simulink model "observer"  (R2020b)
settings: Solver=VariableStepAuto  StartTime=0.0  StopTime=10.0  RelTol=1e-3
settings Model: Creator=10853  LastModifiedBy=10853

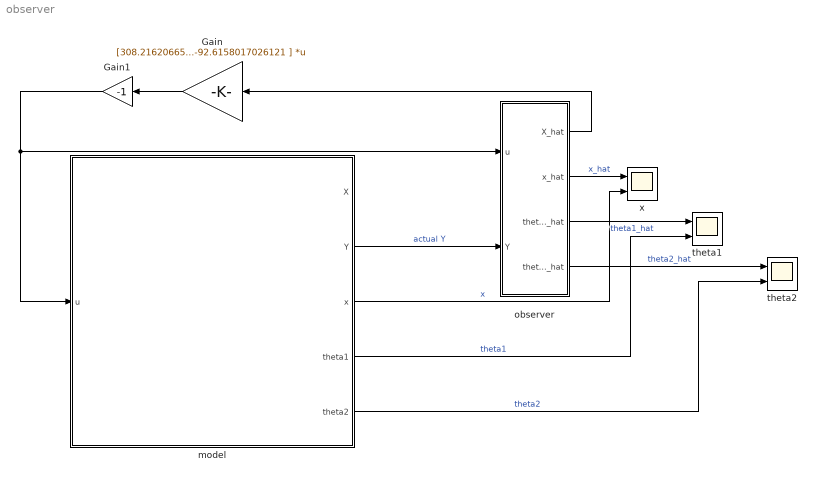
== system observer ==
  Gain : Gain  Gain=|  Multiplication=Matrix(K*u)
      | [308.216206651111	158.619423985671	-617.386289524257	151.829835967496	-19.2479620762821	-92.6158017026121
      | ]
  Gain1 : Gain  Gain=-1
  model : Subsystem
  observer : Subsystem
  theta1 : Scope  NumInputPorts=2
  theta2 : Scope  NumInputPorts=2
  x : Scope  NumInputPorts=2
  wires:
  model/3(x) -> x/2  "x"
  model/4(theta1) -> theta1/2  "theta1"
  model/2(Y) -> observer/2(Y)  "actual Y"
  Gain/1 -> Gain1/1
  Gain1/1 -> model/1(u), observer/1(u)
  observer/2(x_hat) -> x/1  "x_hat"
  observer/3(theta1_hat) -> theta1/1  "theta1_hat"
  model/5(theta2) -> theta2/2  "theta2"
  observer/4(theta2_hat) -> theta2/1  "theta2_hat"
  observer/1(X_hat) -> Gain/1

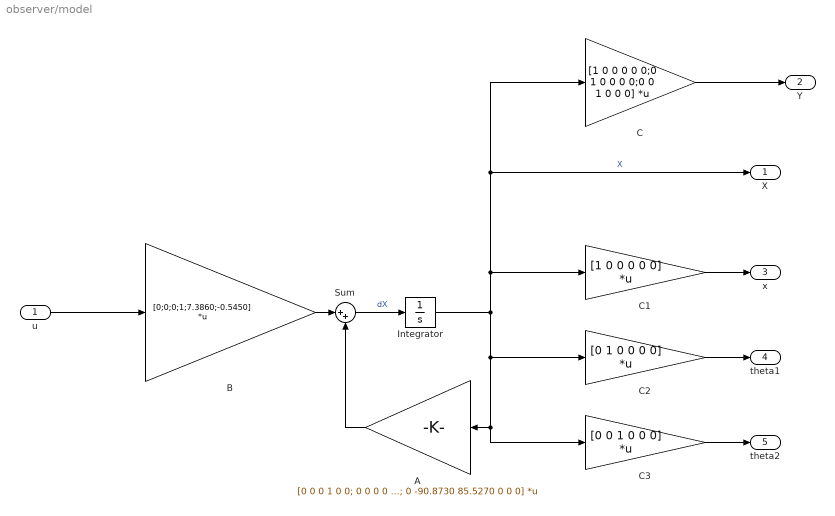
== system observer/model ==
  u : Inport
  A : Gain  Gain=[0 0 0 1 0 0; 0 0 0 0 1 0; 0 0 0 0 0 1;0 0 0 0 0 0; 0 189.318 -116.9320 0 0 0; 0 -90.8730 85.5270 0 0 0]  Multiplication=Matrix(K*u)
  B : Gain  Gain=[0;0;0;1;7.3860;-0.5450]  Multiplication=Matrix(K*u)
  C : Gain  Gain=[1 0 0 0 0 0;0 1 0 0 0 0;0 0 1 0 0 0]  Multiplication=Matrix(K*u)
  C1 : Gain  Gain=[1 0 0 0 0 0]  Multiplication=Matrix(K*u)
  C2 : Gain  Gain=[0 1 0 0 0 0]  Multiplication=Matrix(K*u)
  C3 : Gain  Gain=[0 0 1 0 0 0]  Multiplication=Matrix(K*u)
  Integrator : Integrator  InitialCondition=[0;pi/36;pi/36;0;0;0]
  Sum : Sum  Inputs=|++
  X : Outport
  Y : Outport  Port=2
  x : Outport  Port=3
  theta1 : Outport  Port=4
  theta2 : Outport  Port=5
  wires:
  u/1 -> B/1
  Integrator/1 -> C/1, X/1, C1/1, C2/1, C3/1, A/1  "X"
  C2/1 -> theta1/1
  B/1 -> Sum/1
  A/1 -> Sum/2
  Sum/1 -> Integrator/1  "dX"
  C1/1 -> x/1
  C3/1 -> theta2/1
  C/1 -> Y/1

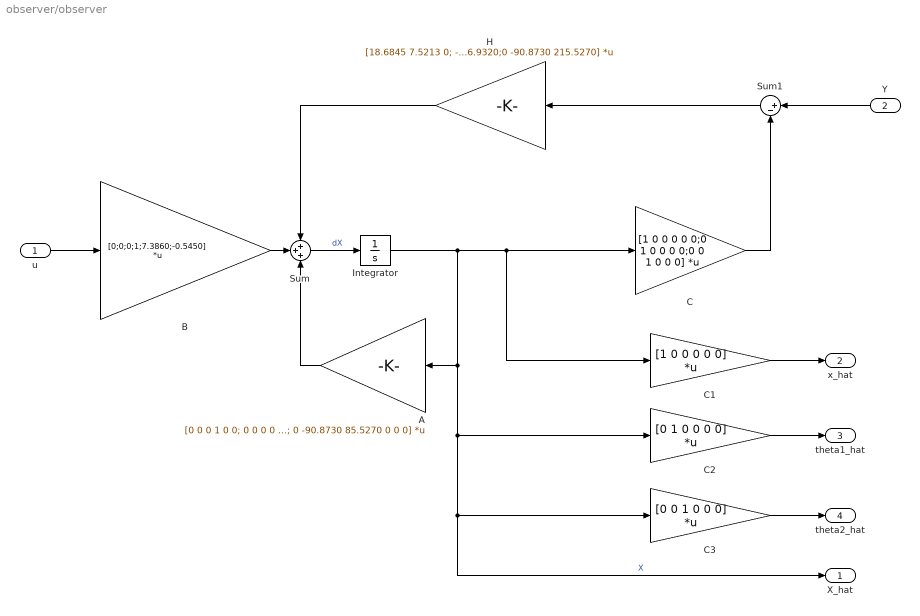
== system observer/observer ==
  u : Inport
  Y : Inport  Port=2
  A : Gain  Gain=[0 0 0 1 0 0; 0 0 0 0 1 0; 0 0 0 0 0 1;0 0 0 0 0 0; 0 189.318 -116.9320 0 0 0; 0 -90.8730 85.5270 0 0 0]  Multiplication=Matrix(K*u)
  B : Gain  Gain=[0;0;0;1;7.3860;-0.5450]  Multiplication=Matrix(K*u)
  C : Gain  Gain=[1 0 0 0 0 0;0 1 0 0 0 0;0 0 1 0 0 0]  Multiplication=Matrix(K*u)
  C1 : Gain  Gain=[1 0 0 0 0 0]  Multiplication=Matrix(K*u)
  C2 : Gain  Gain=[0 1 0 0 0 0]  Multiplication=Matrix(K*u)
  C3 : Gain  Gain=[0 0 1 0 0 0]  Multiplication=Matrix(K*u)
  H : Gain  Gain=[18.6845 7.5213 0; -6.6046 18.4555 0; 0 0 23; 85.2155 83.2607 0; -79.2557 266.7853 -116.9320;0 -90.8730 215.5270]  Multiplication=Matrix(K*u)
  Integrator : Integrator  InitialCondition=[0;0;0;0;0;0]
  Sum : Sum  Inputs=+++
  Sum1 : Sum  Inputs=|+-
  X_hat : Outport
  x_hat : Outport  Port=2
  theta1_hat : Outport  Port=3
  theta2_hat : Outport  Port=4
  wires:
  u/1 -> B/1
  Integrator/1 -> C/1, C1/1, C2/1, C3/1, X_hat/1, A/1  "X"
  C2/1 -> theta1_hat/1
  Sum/1 -> Integrator/1  "dX"
  C1/1 -> x_hat/1
  C3/1 -> theta2_hat/1
  B/1 -> Sum/2
  A/1 -> Sum/3
  H/1 -> Sum/1
  C/1 -> Sum1/2
  Sum1/1 -> H/1
  Y/1 -> Sum1/1
